simulink model "TemporaryHoldingCell"  (R2024b)
settings: Solver=VariableStepAuto  StartTime=0.0  StopTime=10.0  RelTol=1e-3
undefined symbols (not defined in the file): Aero, Motor, Uav
libraries: sharedTrackingLibrary x1
settings Model: Creator=jski306  LastModifiedBy=jski306

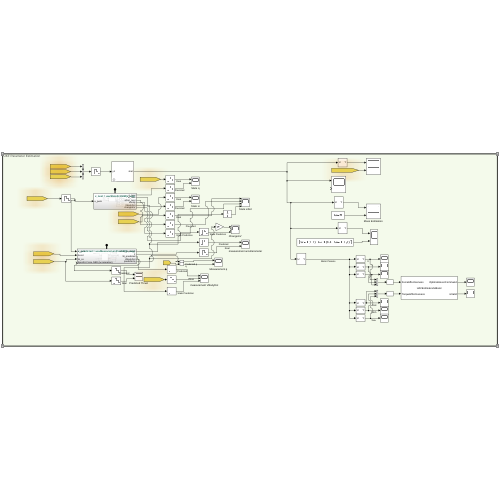
[thumbnail: Simulink's stored preview of the top-level diagram]
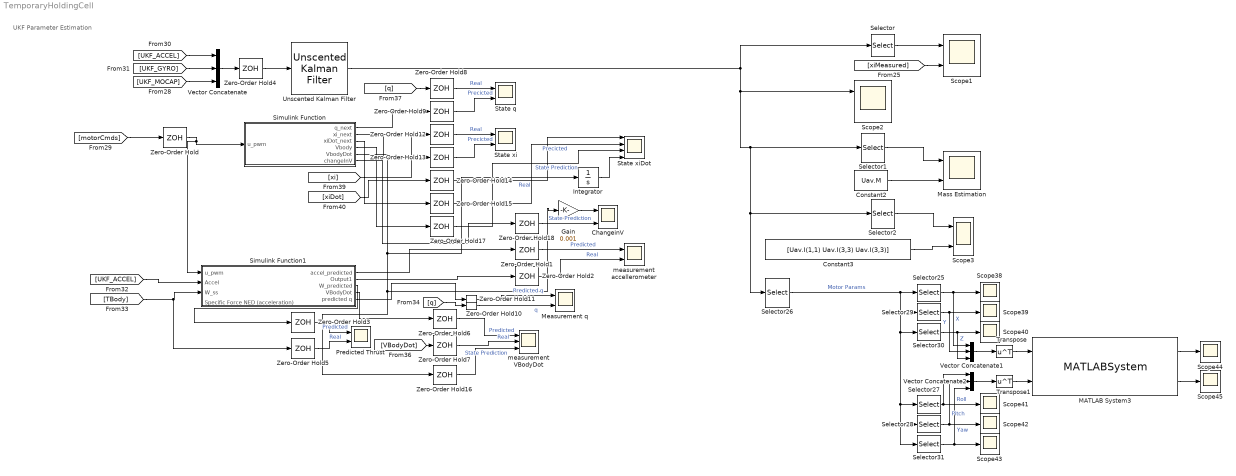
== system TemporaryHoldingCell ==
  note: UKF Parameter Estimation
  ChangeinV : Scope  NumInputPorts=3
  Constant2 : Constant  Value=Uav.M  VectorParams1D=off
  Constant3 : Constant  Value=[Uav.I(1,1) Uav.I(3,3) Uav.I(3,3)]  VectorParams1D=off
  Gain : Gain  Gain=0.001
  Integrator : Integrator
  MATLAB System3 : MATLABSystem  System=UAVEstimateValidator  rotor_count=8  SimulateUsing=Code generation
      mask Type: UAVEstimateValidator
      mask Display:
      | disp('UAVEstimateValidator');
      | port_label('input',1,'ForceEffectiveness');
      | port_label('input',2,'TorqueEffectiveness');
      | port_label('output',1,'OptimalHoverCommand');
      | port_label('output',2,'isValid');
  Mass Estimation : Scope  NumInputPorts=2
  Measurement q : Scope  NumInputPorts=2
  Predicted Thrust : Scope  NumInputPorts=2
  Scope1 : Scope  NumInputPorts=2
  Scope2 : Scope  NumInputPorts=2
  Scope3 : Scope  NumInputPorts=2
  Scope{38..45} (8 alike) : Scope
  Selector : Selector  InputPortWidth=61  IndexOptions=Index vector (dialog)  Indices=[1 2 3]  OutputSizes=1
  Selector1 : Selector  InputPortWidth=61  IndexOptions=Index vector (dialog)  Indices=[14]  OutputSizes=1
  Selector2 : Selector  InputPortWidth=61  IndexOptions=Index vector (dialog)  Indices=[15 16 17]  OutputSizes=1
  Selector25 : Selector  InputPortWidth=48  IndexOptions=Index vector (dialog)  Indices=[1:6:48]  OutputSizes=1
  Selector26 : Selector  InputPortWidth=61  IndexOptions=Index vector (dialog)  Indices=[14:61]  OutputSizes=1
  Selector27 : Selector  InputPortWidth=48  IndexOptions=Index vector (dialog)  Indices=[4:6:48]  OutputSizes=1
  Selector28 : Selector  InputPortWidth=48  IndexOptions=Index vector (dialog)  Indices=[5:6:48]  OutputSizes=1
  Selector29 : Selector  InputPortWidth=48  IndexOptions=Index vector (dialog)  Indices=[2:6:48]  OutputSizes=1
  Selector30 : Selector  InputPortWidth=48  IndexOptions=Index vector (dialog)  Indices=[3:6:48]  OutputSizes=1
  Selector31 : Selector  InputPortWidth=48  IndexOptions=Index vector (dialog)  Indices=[6:6:48]  OutputSizes=1
  Simulink Function : Subsystem  TreatAsAtomicUnit=on
  Simulink Function1 : Subsystem  TreatAsAtomicUnit=on
  State q : Scope  NumInputPorts=2
  State xi : Scope  NumInputPorts=2
  State xiDot : Scope  NumInputPorts=4
  Transpose : Math  Operator=transpose
  Transpose1 : Math  Operator=transpose
  Unscented Kalman Filter : sharedTrackingLibrary/Unscented Kalman Filter  Tag=ParamEstimation  StateTransitionFcn=uavStateFcnSIM  HasAdditiveProcessNoise=Additive  ProcessNoise=UKF.ProcessNoise  HasTimeVaryingProcessNoise=off  HasStateTransitionFcnExtraArgument=0  InitialState=UKF.InitialState  InitialStateCovariance=UKF.InitialCovariance  Alpha=UKF.Alpha  Beta=UKF.Beta  Kappa=UKF.Kappa  MeasurementFcn1=uavMeasurementFcnSIM  HasMeasurementEnablePort1=off  HasAdditiveMeasurementNoise1=Additive  MeasurementNoise1=UKF.MeasurementNoise  HasTimeVaryingMeasurementNoise1=off  HasMeasurementFcnExtraArgument1=0  HasMeasurementWrapping1=off  MeasurementFcn2=myMeasurementFcn  HasMeasurementEnablePort2=off  HasAdditiveMeasurementNoise2=Additive  MeasurementNoise2=1  HasTimeVaryingMeasurementNoise2=off  HasMeasurementFcnExtraArgument2=0  HasMeasurementWrapping2=off  MeasurementFcn3=myMeasurementFcn  HasMeasurementEnablePort3=off  HasAdditiveMeasurementNoise3=Additive  MeasurementNoise3=1  HasTimeVaryingMeasurementNoise3=off  HasMeasurementFcnExtraArgument3=0  HasMeasurementWrapping3=off  MeasurementFcn4=myMeasurementFcn  HasMeasurementEnablePort4=off  HasAdditiveMeasurementNoise4=Additive  MeasurementNoise4=1  HasTimeVaryingMeasurementNoise4=off  HasMeasurementFcnExtraArgument4=0  HasMeasurementWrapping4=off  MeasurementFcn5=myMeasurementFcn  HasMeasurementEnablePort5=off  HasAdditiveMeasurementNoise5=Additive  MeasurementNoise5=1  HasTimeVaryingMeasurementNoise5=off  HasMeasurementFcnExtraArgument5=0  HasMeasurementWrapping5=off  EnableMultirate=off  StateTransitionFcnSampleTime=1  MeasurementFcn1SampleTime=1  MeasurementFcn2SampleTime=1  MeasurementFcn3SampleTime=1  MeasurementFcn4SampleTime=1  MeasurementFcn5SampleTime=1  UseCurrentEstimator=on  OutputStateCovariance=off  DataType=double  SampleTime=0.001  NumberOfMeasurements=1
      settings: LibrarySourceBlock=cstblocks/State Estimation/Unscented Kalman Filter
  Vector Concatenate : Concatenate  NumInputs=3
  Vector Concatenate1 : Concatenate  NumInputs=3  Mode=Multidimensional array  ConcatenateDimension=2
  Vector Concatenate2 : Concatenate  NumInputs=3  Mode=Multidimensional array  ConcatenateDimension=2
  Zero-Order Hold : ZeroOrderHold  SampleTime=0.0001
  Zero-Order Hold{1..3,5..18} (17 alike) : ZeroOrderHold  SampleTime=0.005
  Zero-Order Hold4 : ZeroOrderHold  SampleTime=0.001
  measurement VBodyDot : Scope  NumInputPorts=3
  measurement accellerometer : Scope  NumInputPorts=2
  wires:
  Simulink Function/5(VbodyDot) -> Integrator/1, Gain/1, Zero-Order Hold16/1
  Constant2/1 -> Mass Estimation/2
  Zero-Order Hold4/1 -> Unscented Kalman Filter/1
  Selector28/1 -> Vector Concatenate2/2, Scope42/1  "Pitch"
  Zero-Order Hold13/1 -> State xi/2  "Precicted"
  Vector Concatenate1/1 -> Transpose/1
  Zero-Order Hold7/1 -> measurement VBodyDot/2  "Real"
  Simulink Function1/5(predicted q) -> Zero-Order Hold11/1
  Zero-Order Hold1/1 -> measurement accellerometer/1  "Predicted"
  Zero-Order Hold16/1 -> measurement VBodyDot/3  "State Prediction"
  [q] -> Zero-Order Hold8/1
  [q] -> Zero-Order Hold10/1
  Simulink Function/2(xi_next) -> Zero-Order Hold13/1
  Zero-Order Hold6/1 -> measurement VBodyDot/1  "Predicted"
  Zero-Order Hold18/1 -> ChangeinV/3  "State Prediction"
  Vector Concatenate2/1 -> Transpose1/1
  Selector26/1 -> Selector31/1, Selector28/1, Selector27/1, Selector30/1, Selector29/1, Selector25/1  "Motor Params"
  Zero-Order Hold/1 -> Simulink Function/1(u_pwm), Simulink Function1/1(u_pwm)
  Simulink Function1/2(Output1) -> Zero-Order Hold2/1
  Selector2/1 -> Scope3/1
  Selector/1 -> Scope1/1
  Simulink Function1/1(accel_predicted) -> Zero-Order Hold1/1
  Integrator/1 -> State xiDot/4
  Transpose1/1 -> MATLAB System3/2
  Selector25/1 -> Scope38/1, Vector Concatenate1/1  "X"
  Selector31/1 -> Vector Concatenate2/3, Scope43/1  "Yaw"
  Simulink Function1/4(VBodyDot) -> Zero-Order Hold6/1
  Zero-Order Hold14/1 -> State xiDot/1  "Real"
  Transpose/1 -> MATLAB System3/1
  [motorCmds] -> Zero-Order Hold/1
  [UKF_GYRO] -> Vector Concatenate/2
  [TBody] -> Simulink Function1/3(W_ss), Zero-Order Hold5/1
  Selector27/1 -> Scope41/1, Vector Concatenate2/1  "Roll"
  [xi] -> Zero-Order Hold12/1
  Zero-Order Hold9/1 -> State q/2  "Precicted"
  Selector30/1 -> Vector Concatenate1/3, Scope40/1  "Z"
  Vector Concatenate/1 -> Zero-Order Hold4/1
  Zero-Order Hold5/1 -> Predicted Thrust/2  "Real"
  Simulink Function/1(q_next) -> Zero-Order Hold9/1
  [UKF_ACCEL] -> Simulink Function1/2(Accel)
  Zero-Order Hold2/1 -> measurement accellerometer/2  "Real"
  Simulink Function/4(Vbody) -> Zero-Order Hold17/1
  [xiMeasured] -> Scope1/2
  Selector29/1 -> Scope39/1, Vector Concatenate1/2  "Y"
  Gain/1 -> ChangeinV/1
  [VBodyDot] -> Zero-Order Hold7/1
  Zero-Order Hold17/1 -> State xiDot/3  "State Prediction"
  Constant3/1 -> Scope3/2
  [xiDot] -> Zero-Order Hold14/1
  Simulink Function/6(changeInV) -> Zero-Order Hold18/1
  MATLAB System3/1 -> Scope44/1
  Zero-Order Hold12/1 -> State xi/1  "Real"
  Simulink Function/3(xiDot_next) -> Zero-Order Hold15/1
  Selector1/1 -> Mass Estimation/1
  Simulink Function1/3(W_predicted) -> Zero-Order Hold3/1
  MATLAB System3/2 -> Scope45/1
  Zero-Order Hold8/1 -> State q/1  "Real"
  Unscented Kalman Filter/1 -> Scope2/1, Selector1/1, Selector2/1, Selector26/1, Selector/1
  Zero-Order Hold15/1 -> State xiDot/2  "Precicted"
  Zero-Order Hold3/1 -> Predicted Thrust/1  "Predicted"
  [UKF_MOCAP] -> Vector Concatenate/3
  Zero-Order Hold11/1 -> Measurement q/1  "Predicted q"
  [UKF_ACCEL] -> Vector Concatenate/1
  Zero-Order Hold10/1 -> Measurement q/2  "q"

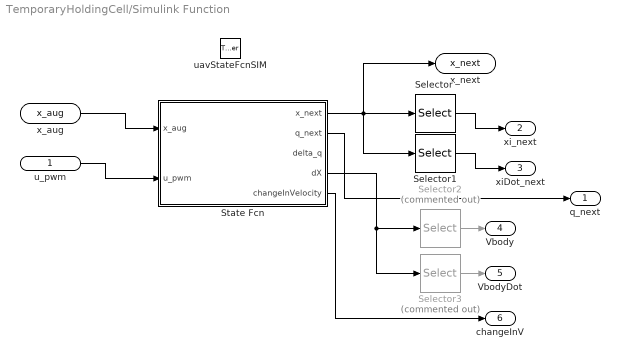
== system TemporaryHoldingCell/Simulink Function ==
  u_pwm : Inport
  uavStateFcnSIM : TriggerPort  TriggerType=function-call  IsSimulinkFunction=on  FunctionName=uavStateFcnSIM  FunctionVisibility=scoped  VariantControl=(inherit)
  Selector : Selector  InputPortWidth=61  IndexOptions=Index vector (dialog)  Indices=[1 2 3]  OutputSizes=1
  Selector1 : Selector  InputPortWidth=61  IndexOptions=Index vector (dialog)  Indices=[4 5 6]  OutputSizes=1
  Selector2 : Selector  Commented=on  InputPortWidth=13  IndexOptions=Index vector (dialog)  Indices=[1 2 3]  OutputSizes=1
  Selector3 : Selector  Commented=on  InputPortWidth=13  IndexOptions=Index vector (dialog)  Indices=[4 5 6]  OutputSizes=1
  State Fcn : MATLAB Function  TreatAsAtomicUnit=on
  x_aug : ArgIn  DisableCoverage=on  PortDimensions=61  ArgumentName=x_aug
  x_next : ArgOut  DisableCoverage=on  PortDimensions=61  ArgumentName=x_next
  q_next : Outport
  xi_next : Outport  Port=2
  xiDot_next : Outport  Port=3
  Vbody : Outport  Port=4
  VbodyDot : Outport  Port=5
  changeInV : Outport  Port=6
  wires:
  x_aug/1 -> State Fcn/1(x_aug)
  State Fcn/1(x_next) -> x_next/1, Selector1/1, Selector/1
  u_pwm/1 -> State Fcn/2(u_pwm)
  Selector/1 -> xi_next/1
  State Fcn/2(q_next) -> q_next/1
  Selector1/1 -> xiDot_next/1
  State Fcn/4(dX) -> Selector3/1, Selector2/1
  Selector2/1 -> Vbody/1
  Selector3/1 -> VbodyDot/1
  State Fcn/5(changeInVelocity) -> changeInV/1

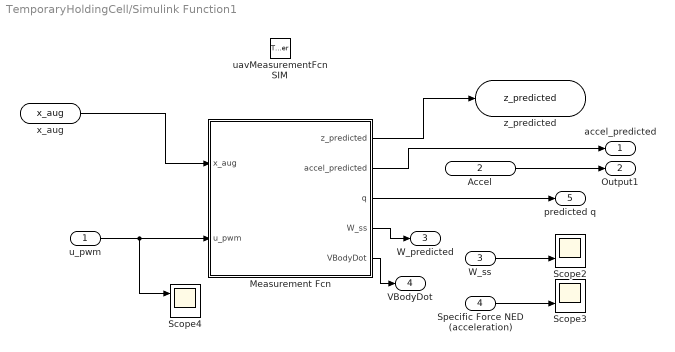
== system TemporaryHoldingCell/Simulink Function1 ==
  u_pwm : Inport
  Accel : Inport  Port=2
  W_ss : Inport  Port=3
  Specific Force NED (acceleration) : Inport  Port=4
  uavMeasurementFcnSIM : TriggerPort  TriggerType=function-call  IsSimulinkFunction=on  FunctionName=uavMeasurementFcnSIM  FunctionVisibility=scoped  VariantControl=(inherit)
  Measurement Fcn : MATLAB Function  TreatAsAtomicUnit=on
  Scope2 : Scope  NumInputPorts=2
  Scope3 : Scope  NumInputPorts=2
  Scope4 : Scope  NumInputPorts=2
  x_aug : ArgIn  DisableCoverage=on  PortDimensions=61  ArgumentName=x_aug
  z_predicted : ArgOut  DisableCoverage=on  PortDimensions=13  ArgumentName=z_predicted
  accel_predicted : Outport
  Output1 : Outport  Port=2
  W_predicted : Outport  Port=3
  VBodyDot : Outport  Port=4
  predicted q : Outport  Port=5
  wires:
  x_aug/1 -> Measurement Fcn/1(x_aug)
  Measurement Fcn/1(z_predicted) -> z_predicted/1
  u_pwm/1 -> Scope4/1, Measurement Fcn/2(u_pwm)
  Measurement Fcn/2(accel_predicted) -> accel_predicted/1
  Accel/1 -> Output1/1
  Measurement Fcn/3(q) -> predicted q/1
  ? -> Scope2/1
  W_ss/1 -> Scope2/2
  Specific Force NED (acceleration)/1 -> Scope3/2
  Measurement Fcn/4(W_ss) -> W_predicted/1
  Measurement Fcn/5(VBodyDot) -> VBodyDot/1

== matlab function TemporaryHoldingCell/Simulink Function/State Fcn ==
  data: x_aug input; x_next output; u_pwm input; Motor parameter; Uav parameter; Aero parameter; q_next output; delta_q output; dX output; changeInVelocity output
function [x_next,q_next,delta_q,dX,changeInVelocity]  = uavStateFcn(x_aug, u_pwm, Motor, Uav, Aero)
%uavStateFcn State transition function using the "Lumped-Parameter" model.

    % --- 1. Unpack Augmented State Vector ---
    dynamic_states = x_aug(1:13);
    
    % --- 2. Define Parameters Structure ---
    % >>>>>>>>>>>> THIS IS THE CRITICAL CHANGE #1 <<<<<<<<<<<<<<<
    % Mass and Inertia are now treated as fixed constants from the Uav struct.
    params.mass    = Uav.M;
    params.Inertia = Uav.I;
    
    % The estimated B-matrix is now unpacked directly from the state vector.
    N_MOTORS = size(u_pwm, 1);
    effectiveness_params = x_aug(14:end);
    B_matrix_estimated = reshape(effectiveness_params, 6, N_MOTORS);
    % -----------------------------------------------------------------

    % Static parameters not included in the estimation
    params.g       = 9.81;
    params.C_tau  = Motor.C_TAU;
    params.Kt     = Motor.K_T;
    params.Ke     = Motor.K_E;
    params.R      = Motor.R;
    params.I0     = Motor.I_0;
    params.V_off  = Motor.Volt_offset;
    params.mv     = Motor.volt_slope;
    
    % >>>>>>>>>>>> THIS IS THE CRITICAL CHANGE #2 <<<<<<<<<<<<<<<
    % The B-matrix is now the estimated parameter from the state.
    % The complex 'for' loop for building the B-matrix is deleted.
    params.B_matrix = B_matrix_estimated;
    
    % --- 3. Call External Helper Functions ---
    W_ss = pwm_to_wrench(u_pwm, params);
    dX   = wrench_to_dynamics_from_sim(dynamic_states, W_ss, params); % accelleration, velocity, ...
    
    % --- 4. Integrate Dynamics Forward ---
    dt = 0.001;
    
    % a) Integrate linear states
    linear_states = [dynamic_states(1:6); dynamic_states(11:13)];
    linear_dX     = [dX(1:6); dX(11:13)];
    changeInVelocity = dt * linear_dX(4:6);
    linear_states_next = linear_states + dt * linear_dX;
    
    % b) Integrate quaternion
    q = dynamic_states(7:10);
    omega = dynamic_states(11:13);
    
    angle = norm(omega) * dt;
    if angle > 1e-6
        axis = omega / norm(omega);
        delta_q = [cos(angle/2); axis(1)*sin(angle/2); axis(2)*sin(angle/2); axis(3)*sin(angle/2)];
    else
        delta_q = [1; 0; 0; 0];
    end
    
    q_next = quaternion_multiply(q, delta_q);
    
    % Safety net for quaternion normalization
    if any(isnan(q_next)) || any(isinf(q_next)) || norm(q_next) < 1e-6
        q_next = [1; 0; 0; 0]; 
    else
        q_next = q_next / norm(q_next);
    end
    
    % --- 5. Assemble the Next Dynamic State ---
    dynamic_states_next = [linear_states_next(1:6); q_next; linear_states_next(7:9)];
    
    % --- 6. Handle Parameter Dynamics ---
    % The parameter dynamics are that they stay constant (random walk).
    params_next = x_aug(14:end);
    
    % --- 7. Assemble the Next Augmented State ---
    x_next = [dynamic_states_next; params_next];
end

% --- LOCAL HELPER FUNCTION ---
function q_out = quaternion_multiply(q1, q2)
    w1 = q1(1); x1 = q1(2); y1 = q1(3); z1 = q1(4);
    w2 = q2(1); x2 = q2(2); y2 = q2(3); z2 = q2(4);
    w = w1*w2 - x1*x2 - y1*y2 - z1*z2;
    x = w1*x2 + x1*w2 + y1*z2 - z1*y2;
    y = w1*y2 - x1*z2 + y1*w2 + z1*x2;
    z = w1*z2 + x1*y2 - y1*x2 + z1*w2;
    q_out = [w; x; y; z];
end

== matlab function TemporaryHoldingCell/Simulink Function1/Measurement Fcn ==
  data: x_aug input; z_predicted output; u_pwm input; Motor parameter; Uav parameter; Aero parameter; accel_predicted output; q output; W_ss output; VBodyDot output
function [z_predicted,accel_predicted,q,W_ss,VBodyDot] = uavMeasurementFcn(x_aug, u_pwm, Motor, Uav, Aero)
%uavMeasurementFcn Predicts sensor readings using the "Lumped-Parameter" model.

    % --- 1. Unpack State Vector ---
    pos_inertial = x_aug(1:3);
    VBody        = x_aug(4:6);
    q            = x_aug(7:10);
    nuBody       = x_aug(11:13);
    
    % >>>>>>>>>>>> THIS IS THE CRITICAL CHANGE #1 <<<<<<<<<<<<<<<
    % Mass and Inertia are now treated as fixed constants from the Uav struct.
    % They are NO LONGER part of the state vector.
    mass         = Uav.M;
    Inertia      = Uav.I;
    g            = 9.81;
    
    % The estimated B-matrix is now unpacked directly from the state vector.
    N_MOTORS = size(u_pwm, 1);
    effectiveness_params = x_aug(14:end);
    B_matrix_estimated = reshape(effectiveness_params, 6, N_MOTORS);
    % -----------------------------------------------------------------

    % --- 2. Predict Gyroscope Reading ---
    gyro_predicted = nuBody;

    % --- 3. Predict Accelerometer Reading (Replicating Plant Model) ---
    % a) Define static parameters
    params.C_tau  = Motor.C_TAU;
    params.Kt     = Motor.K_T;
    params.Ke     = Motor.K_E;
    params.R      = Motor.R;
    params.I0     = Motor.I_0;
    params.V_off  = Motor.Volt_offset;
    params.mv     = Motor.volt_slope;
    
    % b) The B-matrix is now the estimated parameter from the state.
    % >>>>>>>>>>>> THIS IS THE CRITICAL CHANGE #2 <<<<<<<<<<<<<<<
    % The complex 'for' loop for building the B-matrix is deleted.
    params.B_matrix = B_matrix_estimated;
    
    W_ss = pwm_to_wrench(u_pwm, params);
    TBody = W_ss(1:3);

    % c) Calculate gravity's effect in the body frame
    R_b2w = QuatToRot(q);
    R_w2b = R_b2w';
    G_world_NED = [0; 0; g]; 
    G_body = R_w2b * (G_world_NED);

    % d) Calculate VBodyDot using the fixed mass
    VBodyDot  = (TBody/mass) + G_body;

    % e) Rotate VBodyDot into the world (NED) frame
    Accel_NED = (R_b2w * VBodyDot) - G_world_NED;
    
    % f) Final prediction
    accel_predicted = Accel_NED;

    % --- 4. Predict Motion Capture Reading ---
    pos_predicted  = pos_inertial;
    quat_predicted = q;
    mocap_predicted = [pos_predicted; quat_predicted];
    
    % --- 5. Assemble Final Predicted Measurement Vector ---
    z_predicted = [accel_predicted; gyro_predicted; mocap_predicted];
    
    % --- 6. Assign Debug Outputs ---
    % q is already available as a variable.
end

function R = QuatToRot( q )
%QUATTOROT Convert quaternion to rotation matrix
    W = q(1); X = q(2); Y = q(3); Z = q(4);
    xx = X * X; xy = X * Y; xz = X * Z; xw = X * W;
    yy = Y * Y; yz = Y * Z; yw = Y * W;
    zz = Z * Z; zw = Z * W;
    m00 = 1 - 2 * ( yy + zz );
    m01 =     2 * ( xy - zw );
    m02 =     2 * ( xz + yw );
    m10 =     2 * ( xy + zw );
    m11 = 1 - 2 * ( xx + zz );
    m12 =     2 * ( yz - xw );
    m20 =     2 * ( xz - yw );
    m21 =     2 * ( yz + xw );
    m22 = 1 - 2 * ( xx + yy );
    R = [m00 m01 m02; m10 m11 m12; m20 m21 m22];   
end
